simulink model "Model_M1"  (R2018a)
settings: Solver=VariableStepAuto  StartTime=0.0  StopTime=10.0  RelTol=1e-3
libraries: simulink x3
settings Model: Creator=Aniket Raj  LastModifiedBy=Aniket Raj

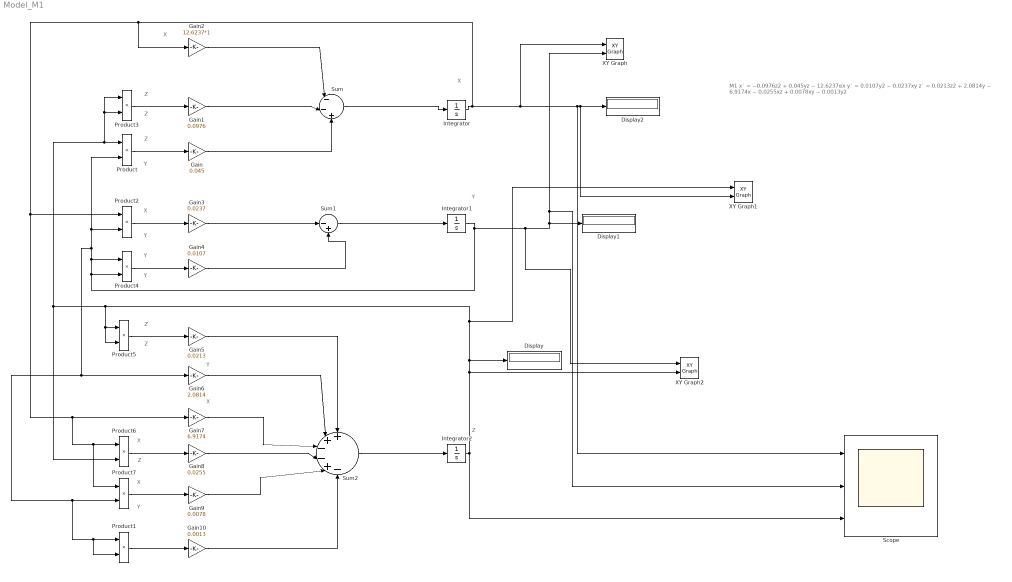
== system Model_M1 ==
  note: Y
  note: X
  note: Z
  note: Z
  note: Y
  note: Z
  note: Y
  note: X
  note: X
  note: Z
  note: Y
  note: Z
  note: Y
  note: Y
  note: Z
  note: Y
  note: X
  note: X
  note: M1
      | x˙ = −0.0976z2 + 0.045yz − 12.6237αx
      | y˙ = 0.0107y2 − 0.0237xy
      | z˙ = 0.0213z2 + 2.0814y − 6.9174x − 0.0255xz + 0.0078xy − 0.0013y2
  note: X
  note: Z
  Display : Display
  Display1 : Display
  Display2 : Display
  Gain : Gain  Gain=0.045
  Gain1 : Gain  Gain=0.0976
  Gain10 : Gain  Gain=0.0013
  Gain2 : Gain  Gain=12.6237*1
  Gain3 : Gain  Gain=0.0237
  Gain4 : Gain  Gain=0.0107
  Gain5 : Gain  Gain=0.0213
  Gain6 : Gain  Gain=2.0814
  Gain7 : Gain  Gain=6.9174
  Gain8 : Gain  Gain=0.0255
  Gain9 : Gain  Gain=0.0078
  Integrator : Integrator  InitialCondition=895.9957
  Integrator1 : Integrator  InitialCondition=2391.688
  Integrator2 : Integrator  InitialCondition=312.7087
  Product{,1..7} (8 alike) : Product
  Scope : Scope  NumInputPorts=3
  Sum : Sum  Inputs=|-|-|+
  Sum1 : Sum  Inputs=|-+
  Sum2 : Sum  Inputs=+|+|-|-|+|-
  XY Graph : simulink/Sinks/XY Graph  xmin=-3000  xmax=3000  ymin=-3000  ymax=3000  st=0.01
  XY Graph1 : simulink/Sinks/XY Graph  xmin=-3000  xmax=3000  ymin=-3000  ymax=3000  st=0.01
  XY Graph2 : simulink/Sinks/XY Graph  xmin=-3000  xmax=3000  ymin=-3000  ymax=3000  st=0.01
  wires:
  Integrator1/1 -> XY Graph2/1, Scope/2, XY Graph/2, Display1/1, Product4/1, Product1/2, Product1/1, Product7/2, Gain6/1, Product2/2, Product/2, Product4/2
  Gain3/1 -> Sum1/1
  Gain8/1 -> Sum2/4
  Integrator/1 -> XY Graph/1, XY Graph1/2, Display2/1, Scope/1, Gain2/1, Product7/1, Product6/1, Gain7/1, Product2/1
  Sum2/1 -> Integrator2/1
  Gain4/1 -> Sum1/2
  Sum1/1 -> Integrator1/1
  Product/1 -> Gain/1
  Gain2/1 -> Sum/1
  Sum/1 -> Integrator/1
  Integrator2/1 -> XY Graph2/2, Display/1, XY Graph1/1, Product3/1, Product3/2, Product/1, Product6/2, Product5/2, Product5/1, Scope/3
  Gain1/1 -> Sum/2
  Product7/1 -> Gain9/1
  Gain6/1 -> Sum2/2
  Gain/1 -> Sum/3
  Product6/1 -> Gain8/1
  Product4/1 -> Gain4/1
  Gain7/1 -> Sum2/3
  Product5/1 -> Gain5/1
  Product3/1 -> Gain1/1
  Product2/1 -> Gain3/1
  Gain5/1 -> Sum2/1
  Gain9/1 -> Sum2/5
  Gain10/1 -> Sum2/6
  Product1/1 -> Gain10/1
